simulink library "csu_pgp_piksi_gps_processing_lib"  (R2014b)
settings: Solver=ode45  StartTime=0.0  StopTime=10.0  RelTol=1e-3
undefined symbols (not defined in the file or in its folder): elk_body_base_to_origin, elk_launchstand_height
libraries: simulink x3, util_common_lib x3, util_event_lib x2, csu_und_unduplicate_lib x2, util_info_lib x1
settings Model: Creator=escrane  LastModifiedBy=tgorton

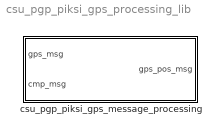
== system csu_pgp_piksi_gps_processing_lib ==
  csu_pgp_piksi_gps_message_processing : Subsystem

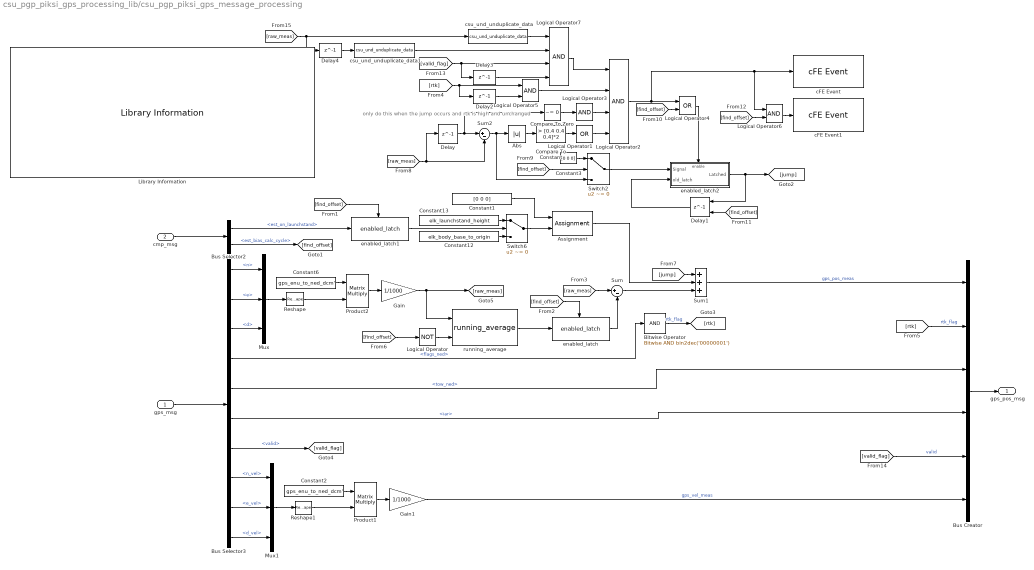
== system csu_pgp_piksi_gps_processing_lib/csu_pgp_piksi_gps_message_processing ==
  note: only do this when the jump occurs and rtk is high and unchanged
  gps_msg : Inport
  cmp_msg : Inport  Port=2
  Abs : Abs
  Assignment : Assignment  DiagnosticForDimensions=Warning  Indices=3
  Bitwise Operator : simulink/Logic and Bit Operations/Bitwise Operator  logicop=AND  UseBitMask=on  BitMask=bin2dec('00000001')  BitMaskRealWorld=Stored Integer
  Bus Creator : BusCreator  Inputs=6
  Bus Selector2 : BusSelector  OutputSignals=est_on_launchstand,est_bias_calc_cycle
  Bus Selector3 : BusSelector  OutputSignals=n,e,d,flags_ned,tow_ned,iar,valid,n_vel,e_vel,d_vel
  Compare To Constant : simulink/Logic and Bit Operations/Compare To Constant  relop=>  const=[0.4 0.4 0.4]*2  OutDataTypeStr=boolean
  Compare To Zero : simulink/Logic and Bit Operations/Compare To Zero  relop=~=  OutDataTypeStr=boolean
  Constant1 : Constant  Value=[0 0 0]  OutDataTypeStr=double
  Constant12 : Constant  Value=elk_body_base_to_origin  VectorParams1D=off
  Constant13 : Constant  Value=elk_launchstand_height  VectorParams1D=off
  Constant2 : Constant  Value=gps_enu_to_ned_dcm'
  Constant3 : Constant  Value=[0 0 0]  OutDataTypeStr=double
  Constant6 : Constant  Value=gps_enu_to_ned_dcm'
  Delay{,2..4} (4 alike) : Delay  DelayLength=1  InitialCondition=0
  Delay1 : Delay  DelayLength=1  InitialCondition=0  ExternalReset=Rising
      settings: InputPortMap=u0,r5
  Gain : Gain  Gain=1/1000
  Gain1 : Gain  Gain=1/1000
  Library Information : util_info_lib/Library Information  owner='escrane'
  Logical Operator : Logic  Operator=NOT  AllPortsSameDT=off  OutDataTypeStr=boolean
  Logical Operator1 : Logic  Operator=OR  Inputs=1  AllPortsSameDT=off  OutDataTypeStr=boolean
  Logical Operator2 : Logic  Inputs=4  AllPortsSameDT=off  OutDataTypeStr=boolean
  Logical Operator3 : Logic  Inputs=1  AllPortsSameDT=off  OutDataTypeStr=boolean
  Logical Operator4 : Logic  Operator=OR  AllPortsSameDT=off  OutDataTypeStr=boolean
  Logical Operator5 : Logic  AllPortsSameDT=off  OutDataTypeStr=boolean
  Logical Operator6 : Logic  AllPortsSameDT=off  OutDataTypeStr=boolean
  Logical Operator7 : Logic  Inputs=4  AllPortsSameDT=off  OutDataTypeStr=boolean
  Mux : Mux  Inputs=3
  Mux1 : Mux  Inputs=3
  Product1 : Product  Multiplication=Matrix(*)
  Product2 : Product  Multiplication=Matrix(*)
  Reshape : Reshape  OutputDimensionality=Column vector (2-D)
  Reshape1 : Reshape  OutputDimensionality=Column vector (2-D)
  Sum : Sum  Inputs=|+-
  Sum1 : Sum  Inputs=+++
  Sum2 : Sum  Inputs=|+-
  Switch2 : Switch  Criteria=u2 ~= 0  Threshold=0.5  InputSameDT=on
  Switch6 : Switch  Criteria=u2 ~= 0  Threshold=0.5  InputSameDT=on
  cFE Event : util_event_lib/cFE Event  event_message='GPS measurement has jumped. Absorbing in offset calculation.'  event_id=45  event_severity=INFORMATION  event_filtered=off  event_mask=1  event_use_enums=off  event_enum_types={}
  cFE Event1 : util_event_lib/cFE Event  event_message='ALERT: GPS measurement has jumped while calculating offset.'  event_id=45  event_severity=ERROR  event_filtered=off  event_mask=1  event_use_enums=off  event_enum_types={}
  csu_und_unduplicate_data : csu_und_unduplicate_lib/csu_und_unduplicate_data  initial_compare=0
  csu_und_unduplicate_data1 : csu_und_unduplicate_lib/csu_und_unduplicate_data  initial_compare=0
  enabled_latch : util_common_lib/enabled_latch  initial_output=0
  enabled_latch1 : util_common_lib/enabled_latch  initial_output=cml_initial_value.est_on_launchstand
  enabled_latch2 : Subsystem  mask{initial_output=0}
      mask prompts: initial_output "Initial Output Value"
      mask Display:
      | color('blue')
      | text(0.05,0.02,'NASA',...
      |  	'HorizontalAlignment','Left',...
      | 	'VerticalAlignment','bottom')
  running_average : util_common_lib/running_average  initial_mean=[0 0 0]'
  gps_pos_msg : Outport
  wires:
  Gain1/1 -> Bus Creator/6  "gps_vel_meas"
  Delay4/1 -> csu_und_unduplicate_data1/1
  csu_und_unduplicate_data1/1 -> Logical Operator7/2
  csu_und_unduplicate_data/1 -> Logical Operator7/1
  [raw_meas] -> csu_und_unduplicate_data/1, Delay4/1
  [valid_flag] -> Bus Creator/5  "valid"
  [valid_flag] -> Delay3/1, Logical Operator7/3
  Delay3/1 -> Logical Operator7/4
  Logical Operator7/1 -> Logical Operator2/1
  Product1/1 -> Gain1/1
  Reshape1/1 -> Product1/2
  Constant2/1 -> Product1/1
  Mux1/1 -> Reshape1/1
  Bus Selector3/10 -> Mux1/3  "<d_vel>"
  Bus Selector3/9 -> Mux1/2  "<e_vel>"
  Bus Selector3/8 -> Mux1/1  "<n_vel>"
  [find_offset] -> Logical Operator6/2
  Logical Operator6/1 -> cFE Event1/1
  Assignment/1 -> Sum1/2
  [jump] -> Sum1/1
  Bitwise Operator/1 -> [rtk]  "rtk_flag"
  [raw_meas] -> Sum/1
  [raw_meas] -> Delay/1, Sum2/2
  Logical Operator5/1 -> Logical Operator2/2
  Delay2/1 -> Logical Operator5/2
  [rtk] -> Logical Operator5/1, Delay2/1
  [find_offset] -> Delay1/2
  Logical Operator4/1 -> enabled_latch2/Enable
  [find_offset] -> Logical Operator4/2
  Logical Operator2/1 -> Logical Operator4/1, cFE Event/1, Logical Operator6/1
  Switch2/1 -> enabled_latch2/1(Signal)
  Constant3/1 -> Switch2/1
  [find_offset] -> Switch2/2
  enabled_latch2/1(Latched) -> [jump], Delay1/1
  Delay1/1 -> enabled_latch2/2(old_latch)
  Compare To Zero/1 -> Logical Operator3/1
  Logical Operator3/1 -> Logical Operator2/3
  Logical Operator1/1 -> Logical Operator2/4
  Compare To Constant/1 -> Logical Operator1/1
  Abs/1 -> Compare To Constant/1
  Sum2/1 -> Switch2/3, Abs/1
  Delay/1 -> Sum2/1, Compare To Zero/1
  Bus Selector3/7 -> [valid_flag]  "<valid>"
  Bus Selector2/2 -> [find_offset]  "<est_bias_calc_cycle>"
  Sum1/1 -> Bus Creator/1  "gps_pos_meas"
  Bus Selector3/6 -> Bus Creator/4  "<iar>"
  Bus Selector3/5 -> Bus Creator/3  "<tow_ned>"
  [find_offset] -> enabled_latch/Enable
  [find_offset] -> enabled_latch1/Enable
  Bus Selector2/1 -> enabled_latch1/1  "<est_on_launchstand>"
  enabled_latch1/1 -> Switch6/2
  Constant1/1 -> Assignment/1
  Switch6/1 -> Assignment/2
  Constant12/1 -> Switch6/3
  Constant13/1 -> Switch6/1
  cmp_msg/1 -> Bus Selector2/1
  Sum/1 -> Sum1/3
  [rtk] -> Bus Creator/2  "rtk_flag"
  Logical Operator/1 -> running_average/2
  [find_offset] -> Logical Operator/1
  running_average/1 -> enabled_latch/1
  enabled_latch/1 -> Sum/2
  Bus Creator/1 -> gps_pos_msg/1
  Bus Selector3/4 -> Bitwise Operator/1  "<flags_ned>"
  Gain/1 -> running_average/1, [raw_meas]
  Product2/1 -> Gain/1
  Reshape/1 -> Product2/2
  Constant6/1 -> Product2/1
  Mux/1 -> Reshape/1
  Bus Selector3/3 -> Mux/3  "<d>"
  Bus Selector3/2 -> Mux/2  "<e>"
  Bus Selector3/1 -> Mux/1  "<n>"
  gps_msg/1 -> Bus Selector3/1

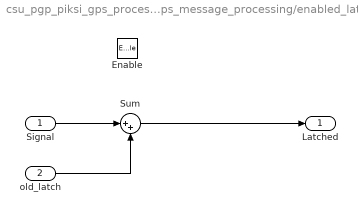
== system csu_pgp_piksi_gps_processing_lib/csu_pgp_piksi_gps_message_processing/enabled_latch2 ==
  Signal : Inport
  old_latch : Inport  Port=2
  Enable : EnablePort
  Sum : Sum  Inputs=|++
  Latched : Outport  InitialOutput=initial_output
  wires:
  old_latch/1 -> Sum/2
  Sum/1 -> Latched/1
  Signal/1 -> Sum/1
